simulink model "Workshop_as_sim_part2"  (Simulink 9.3)
settings: Solver=ode1  StartTime=0.0  StopTime=50  FixedStep=0.001  RelTol=1e-3  EnableMultiTasking=on
PostLoadFcn:
  | qc_set_target_type(getConfigSet(bdroot, 'QUARC Default Target Configuration'));
undefined symbols (not defined in the file or in its folder): actuator_pnoise_pow, actuator_tf_den, actuator_tf_num, anom_set_size, HIL, input_delay_length, qc_get_step_size, tire_mnoise_pow, use_actuator_pnoise, use_input_delay, use_roadpos_anomalies, use_roadpos_noise, use_tire_mnoise, use_vb_mnoise, vb_mnoise_pow
libraries: quarc_library x8, simulink x6, commrandsrc3 x1
settings Model: Creator=DCrymble  LastModifiedBy=jxs210080  SimulationMode=external  ExtModeTrigDuration=50000
settings SolverCC: PositivePriorityOrder=on
settings DataIOCC: LimitDataPoints=on
settings OptimizationCC: ExpressionDepthLimit=2147483647  InitFltsAndDblsToZero=on  LifeSpan=auto
settings DebuggingCC: SaveWithParameterizedLinksMsg=none  SolverPrmCheckMsg=warning  MultiTaskDSMMsg=warning  MultiTaskCondExecSysMsg=none  StateNameClashWarn=warning
settings RTWCC: SystemTargetFile=quarc_win64.tlc  TemplateMakefile=quarc_default_tmf  Description=QUARC Win64 Target
settings STFCustomTargetCC: TargetPreCompLibLocation=C:\PROGRA~3\QUARC\lib\2019a\win64\release  ConcurrentExecutionCompliant=on  SystemTargetFile=quarc_win64.tlc
settings GRTTargetCC: TargetPreCompLibLocation=C:\PROGRA~3\QUARC\lib\2019a\win64\release  ParMdlRefBuildCompliant=off  CompOptLevelCompliant=off  MatFileLogging=off  CPPClassGenCompliant=off  UseToolchainInfoCompliant=off  ExtMode=on  ExtModeMexFile=quarc_comm
settings ConfigComp: CovHtmlReporting=off

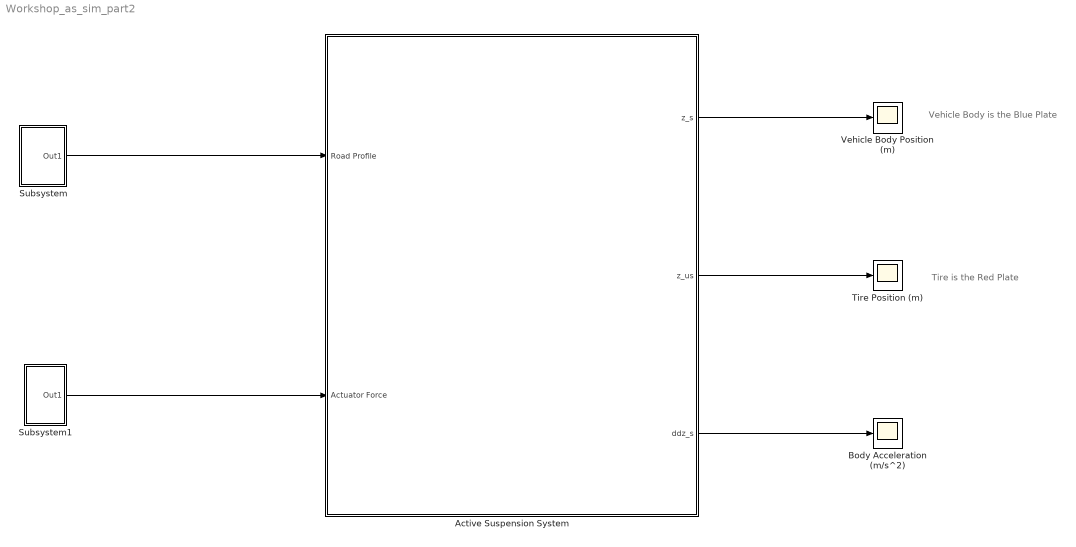
== system Workshop_as_sim_part2 ==
  note: Vehicle Body is the Blue Plate
  note: Tire is the Red Plate
  Active Suspension System : Subsystem
      mask Display: image('icon.png');
  Body Acceleration (m/s^2) : Scope
  Subsystem : Subsystem
  Subsystem1 : Subsystem
  Tire Position (m) : Scope
  Vehicle Body Position (m) : Scope
  wires:
  Active Suspension System/3(ddz_s) -> Body Acceleration (m/s^2)/1
  Active Suspension System/2(z_us) -> Tire Position (m)/1
  Active Suspension System/1(z_s) -> Vehicle Body Position (m)/1
  Subsystem/1(Out1) -> Active Suspension System/1(Road Profile)
  Subsystem1/1(Out1) -> Active Suspension System/2(Actuator Force)

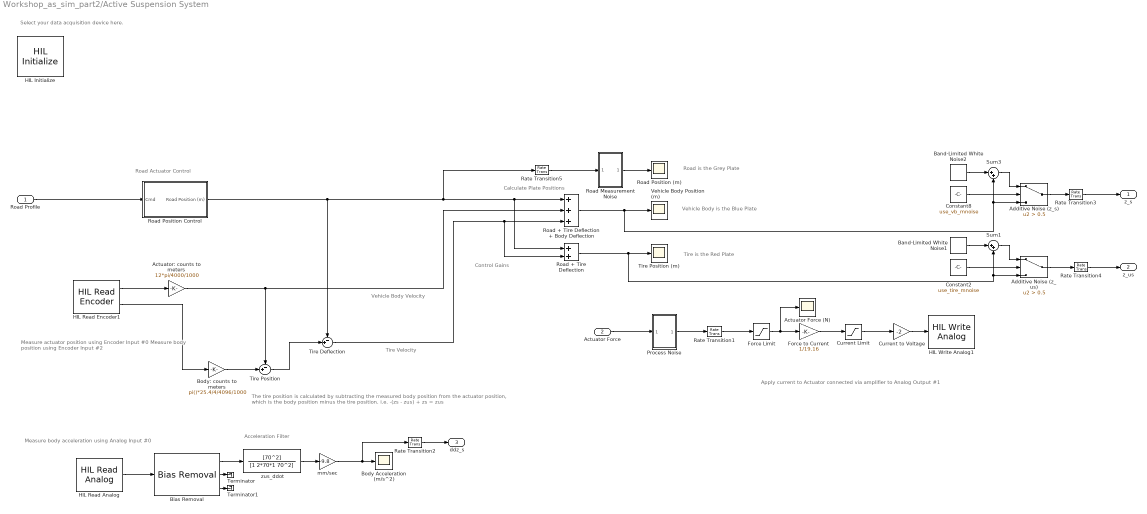
== system Workshop_as_sim_part2/Active Suspension System ==
  note: Measure actuator position using Encoder Input  #0
      | Measure body position using Encoder Input #2
  note: Select your data acquisition device here.
  note: Control Gains
  note: Vehicle Body Velocity
  note: Tire Velocity
  note: Road Actuator Control
  note: Calculate Plate Positions
  note: Measure body acceleration using Analog Input #0
  note: Acceleration Filter
  note: Apply current to Actuator connected via amplifier to Analog Output #1
  note: Road is the Grey Plate
  note: Vehicle Body is the Blue Plate
  note: Tire is the Red Plate
  note: The tire position is calculated by subtracting the measured body position from
      | the actuator position, which is the body position minus the tire position.
      | i.e. -(zs - zus) + zs = zus
  Road Profile : Inport
  Actuator Force : Inport  Port=2
  Actuator Force (N) : Scope
  Actuator: counts to meters : Gain  Gain=12*pi/4000/1000
  Additive Noise (z_s) : Switch  Criteria=u2 > Threshold  Threshold=0.5
  Additive Noise (z_us) : Switch  Criteria=u2 > Threshold  Threshold=0.5
  Band-Limited White Noise1 : simulink/Sources/Band-Limited White Noise  Cov=[tire_mnoise_pow]  Ts=0.001  seed=[23341]
  Band-Limited White Noise2 : simulink/Sources/Band-Limited White Noise  Cov=[vb_mnoise_pow]  Ts=0.001  seed=[23341]
  Bias Removal : quarc_library/Discrete/Bias Removal  start_time=0  end_time=.099  switch_id=0  sample_time=qc_get_step_size
      settings: SourceProductName=QUARC Targets
  Body Acceleration (m/s^2) : Scope
  Body: counts to meters : Gain  Gain=pi()*25.4/4/4096/1000
  Constant2 : Constant  Value=use_tire_mnoise
  Constant8 : Constant  Value=use_vb_mnoise
  Current Limit : Saturate  UpperLimit=5  LowerLimit=-5
  Current to Voltage : Gain  Gain=-2
  Force Limit : Saturate  UpperLimit=39.2  LowerLimit=-39.2
  Force to Current : Gain  Gain=1/19.16
  HIL Initialize : quarc_library/Data Acquisition/Generic/Configuration/HIL Initialize  Priority=-99  object_name=HIL-1  board_type=q8_usb  board_number=0  board_options=update_rate=normal;decimation=1  exclusive=off  active=off  hardware_clocks=[0:2]  clock_modes=[]  initial_clock_frequencies=[]  set_clock_params_at_start=off  set_clock_params_at_switch_in=off  set_clock_frequencies_at_start=off  set_clock_frequencies_at_switch_in=off  analog_input_channels=[0:7]  analog_input_configurations=[]  analog_input_maximums=10  analog_input_minimums=-10  set_analog_input_params_at_start=on  set_analog_input_params_at_switch_in=off  analog_output_channels=[0:7]  analog_output_maximums=10  analog_output_minimums=-10  initial_analog_outputs=[0]  final_analog_outputs=[0]  watchdog_analog_outputs=0  set_analog_output_params_at_start=on  set_analog_output_params_at_switch_in=off  set_analog_outputs_at_start=on  set_analog_outputs_at_switch_in=off  set_analog_outputs_at_terminate=on  set_analog_outputs_at_switch_out=off  set_analog_outputs_on_watchdog=off  digital_input_channels=[]  digital_output_channels=[0:4]  digital_output_configuration=[]  initial_digital_outputs=[0 0 0 0 1]  final_digital_outputs=[1 1 1 1 0]  watchdog_digital_outputs=[0]  set_digital_output_params_at_start=off  set_digital_output_params_at_switch_in=off  set_digital_outputs_at_start=on  set_digital_outputs_at_switch_in=on  set_digital_outputs_at_terminate=on  set_digital_outputs_at_switch_out=off  set_digital_outputs_on_watchdog=off  encoder_channels=[0:7]  quadrature=[4]  encoder_filter_frequency=[]  initial_encoder_counts=[0]  set_encoder_params_at_start=on  set_encoder_params_at_switch_in=off  set_encoder_counts_at_start=on  set_encoder_counts_at_switch_in=off  pwm_channels=[0:7]  pwm_modes=0  pwm_frequency=99.532799999999995e6/4095  pwm_configuration=[0]  pwm_alignment=[0]  pwm_polarity=[1]  pwm_leading_deadband=[0]  pwm_trailing_deadband=[0]  initial_pwm_outputs=[0]  final_pwm_outputs=[0]  watchdog_pwm_outputs=[0]  set_pwm_params_at_start=on  set_pwm_params_at_switch_in=off  set_pwm_outputs_at_start=on  set_pwm_outputs_at_switch_in=off  set_pwm_outputs_at_terminate=on  set_pwm_outputs_at_switch_out=off  set_pwm_outputs_on_watchdog=off  other_output_channels=[]  initial_other_outputs=[]  final_other_outputs=[]  watchdog_other_outputs=[]  set_other_outputs_at_start=off  set_other_outputs_at_switch_in=off  set_other_outputs_at_terminate=off  set_other_outputs_at_switch_out=off  set_other_outputs_on_watchdog=off
  HIL Read Analog : quarc_library/Data Acquisition/Generic/Immediate I//O/HIL Read Analog  object_name=HIL-1  channels=0  sample_time=qc_get_step_size  active=on  vector_output=off
  HIL Read Encoder1 : quarc_library/Data Acquisition/Generic/Immediate I//O/HIL Read Encoder  object_name=HIL-1  channels=[0, 2]  sample_time=qc_get_step_size  active=on  vector_output=off  data_type_mode=Inherit via back propagation  data_type=double
  HIL Write Analog1 : quarc_library/Data Acquisition/Generic/Immediate I//O/HIL Write Analog  object_name=HIL-1  channels=0  sample_time=-1  active=off  vector_input=on
  "Process Noise " : Subsystem
  Rate Transition1 : RateTransition  OutPortSampleTime=0.1
  Rate Transition{2..5} (4 alike) : RateTransition  OutPortSampleTime=0.01
  Road + Tire Deflection : Sum  Inputs=2  SaturateOnIntegerOverflow=on  InputSameDT=on  OutDataTypeStr=Inherit: Same as first input
  Road + Tire Deflection + Body Deflection : Sum  Inputs=3  SaturateOnIntegerOverflow=on  InputSameDT=on  OutDataTypeStr=Inherit: Same as first input
  Road Measurement Noise : Subsystem
  Road Position (m) : Scope
  Road Position Control : Subsystem
  Sum1 : Sum  Inputs=|++
  Sum3 : Sum  Inputs=|++
  Terminator : Terminator
  Terminator1 : Terminator
  Tire Deflection : Sum  Inputs=-+|
  Tire Position : Sum  Inputs=-+|
  Tire Position (m) : Scope
  Vehicle Body Position (m) : Scope
  mm/sec : Gain  Gain=-9.8
  zus_ddot : TransferFcn  Numerator=[70^2]  Denominator=[1 2*70*1 70^2]
  z_s : Outport
  z_us : Outport  Port=2
  ddz_s : Outport  Port=3
  wires:
  HIL Read Encoder1/1 -> Actuator: counts to meters/1
  Tire Deflection/1 -> Road + Tire Deflection + Body Deflection/3, Road + Tire Deflection/2
  HIL Read Encoder1/2 -> Body: counts to meters/1
  Body: counts to meters/1 -> Tire Position/2
  Road Position Control/1(Road Position (m)) -> Tire Deflection/1, Road + Tire Deflection + Body Deflection/1, Road + Tire Deflection/1, Rate Transition5/1
  Tire Position/1 -> Tire Deflection/2
  Bias Removal/2 -> Terminator/1
  Current to Voltage/1 -> HIL Write Analog1/1
  Force to Current/1 -> Current Limit/1
  Road Profile/1 -> Road Position Control/1(Cmd)
  Force Limit/1 -> Actuator Force (N)/1, Force to Current/1
  zus_ddot/1 -> mm/sec/1
  mm/sec/1 -> Rate Transition2/1, Body Acceleration (m/s^2)/1
  Bias Removal/1 -> zus_ddot/1
  Current Limit/1 -> Current to Voltage/1
  HIL Read Analog/1 -> Bias Removal/1
  Bias Removal/3 -> Terminator1/1
  Actuator Force/1 -> "Process Noise "/1(In1)
  Rate Transition2/1 -> ddz_s/1
  Rate Transition4/1 -> z_us/1
  Rate Transition3/1 -> z_s/1
  Rate Transition1/1 -> Force Limit/1
  Road + Tire Deflection + Body Deflection/1 -> Vehicle Body Position (m)/1, Sum3/2, Additive Noise (z_s)/3
  Additive Noise (z_s)/1 -> Rate Transition3/1
  Sum3/1 -> Additive Noise (z_s)/1
  Band-Limited White Noise2/1 -> Sum3/1
  Constant8/1 -> Additive Noise (z_s)/2
  Constant2/1 -> Additive Noise (z_us)/2
  Band-Limited White Noise1/1 -> Sum1/1
  Sum1/1 -> Additive Noise (z_us)/1
  Additive Noise (z_us)/1 -> Rate Transition4/1
  Road + Tire Deflection/1 -> Sum1/2, Additive Noise (z_us)/3, Tire Position (m)/1
  Actuator: counts to meters/1 -> Tire Position/1, Road + Tire Deflection + Body Deflection/2
  Road Measurement Noise/1(Out1) -> Road Position (m)/1
  "Process Noise "/1(Out1) -> Rate Transition1/1
  Rate Transition5/1 -> Road Measurement Noise/1(In1)

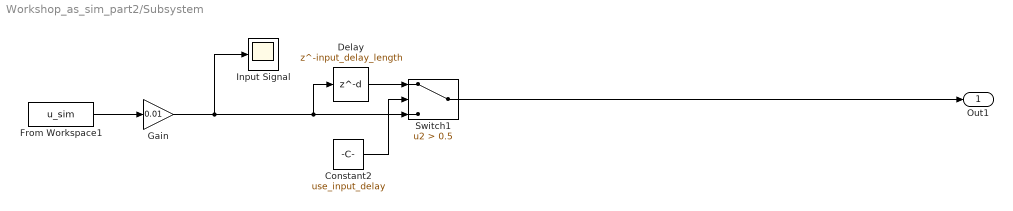
== system Workshop_as_sim_part2/Subsystem ==
  Constant2 : Constant  Value=use_input_delay
  Delay : Delay  DelayLength=input_delay_length
  From Workspace1 : FromWorkspace  VariableName=u_sim  SampleTime=0.01
  Gain : Gain  Gain=0.01
  Input Signal : Scope
  Switch1 : Switch  Criteria=u2 > Threshold  Threshold=0.5
  Out1 : Outport
  wires:
  Switch1/1 -> Out1/1
  From Workspace1/1 -> Gain/1
  Gain/1 -> Input Signal/1, Delay/1, Switch1/3
  Delay/1 -> Switch1/1
  Constant2/1 -> Switch1/2

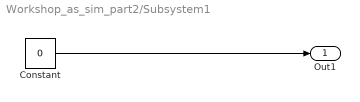
== system Workshop_as_sim_part2/Subsystem1 ==
  Constant : Constant  Value=0
  Out1 : Outport
  wires:
  Constant/1 -> Out1/1

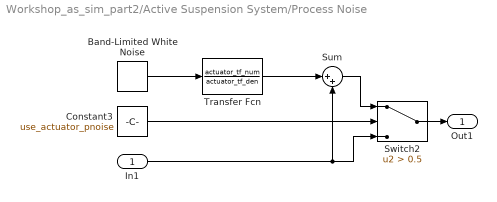
== system Workshop_as_sim_part2/Active Suspension System/Process Noise  ==
  In1 : Inport
  Band-Limited White Noise : simulink/Sources/Band-Limited White Noise  Cov=[actuator_pnoise_pow]  Ts=0.001  seed=[23341]
  Constant3 : Constant  Value=use_actuator_pnoise
  Sum : Sum  Inputs=|++
  Switch2 : Switch  Criteria=u2 > Threshold  Threshold=0.5
  Transfer Fcn : TransferFcn  Numerator=actuator_tf_num  Denominator=actuator_tf_den
  Out1 : Outport
  wires:
  Band-Limited White Noise/1 -> Transfer Fcn/1
  In1/1 -> Switch2/3, Sum/2
  Transfer Fcn/1 -> Sum/1
  Constant3/1 -> Switch2/2
  Sum/1 -> Switch2/1
  Switch2/1 -> Out1/1

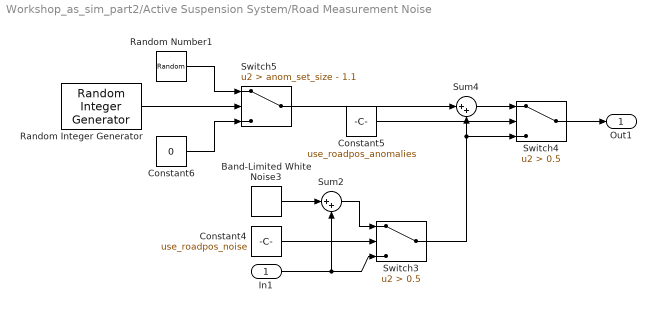
== system Workshop_as_sim_part2/Active Suspension System/Road Measurement Noise ==
  In1 : Inport
  Band-Limited White Noise3 : simulink/Sources/Band-Limited White Noise  Cov=roadpos_noise_pow  Ts=0.01  seed=[23341]
  Constant4 : Constant  Value=use_roadpos_noise
  Constant5 : Constant  Value=use_roadpos_anomalies
  Constant6 : Constant  Value=0
  Random Number1 : RandomNumber  Variance=100  SampleTime=0.01
  Random Integer Generator : commrandsrc3/Random Integer Generator  SetSize=anom_set_size  SeedSource=Auto  Seed=0  SampleTime=0.01  SamplesPerFrame=1  OutputDataType=double  SimulateUsing=Interpreted execution
      settings: SourceProductName=Communications Toolbox
  Sum2 : Sum  Inputs=|++
  Sum4 : Sum  Inputs=|++
  Switch3 : Switch  Criteria=u2 > Threshold  Threshold=0.5
  Switch4 : Switch  Criteria=u2 > Threshold  Threshold=0.5
  Switch5 : Switch  Criteria=u2 > Threshold  Threshold=anom_set_size - 1.1
  Out1 : Outport
  wires:
  Band-Limited White Noise3/1 -> Sum2/1
  Switch5/1 -> Sum4/1
  Random Integer Generator/1 -> Switch5/2
  Constant4/1 -> Switch3/2
  Constant5/1 -> Switch4/2
  Random Number1/1 -> Switch5/1
  Sum4/1 -> Switch4/1
  Switch3/1 -> Switch4/3, Sum4/2
  Constant6/1 -> Switch5/3
  In1/1 -> Sum2/2, Switch3/3
  Sum2/1 -> Switch3/1
  Switch4/1 -> Out1/1

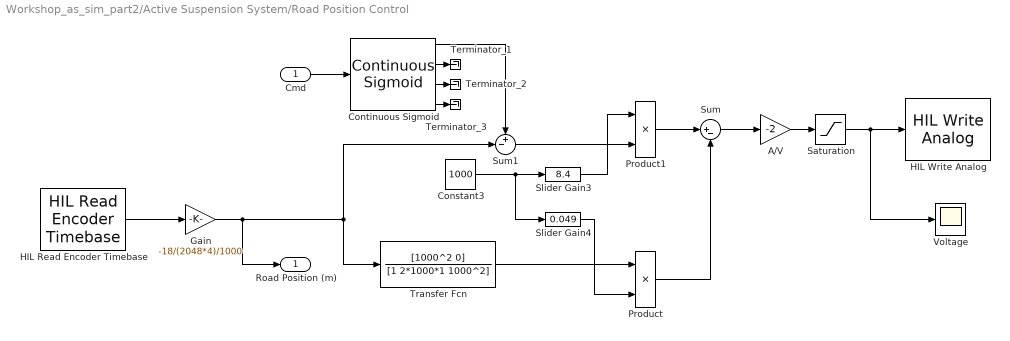
== system Workshop_as_sim_part2/Active Suspension System/Road Position Control ==
  Cmd : Inport
  A/V : Gain  Gain=-2
  Constant3 : Constant  Value=1000
  Continuous Sigmoid : quarc_library/Sources/Sigmoids/Continuous Sigmoid  params_source=Internal (dialog parameters)  max_velocity=.6/3  max_acceleration=20  initial_position=0  initial_velocity=0  hold_off=0.5  input_sample_time=-1  output_sample_time=qc_get_step_size
      settings: SourceProductName=QUARC Targets
  Gain : Gain  Gain=-18/(2048*4)/1000
  HIL Read Encoder Timebase : quarc_library/Data Acquisition/Generic/Timebases/HIL Read Encoder Timebase  object_name=HIL-1  clock=[0]  channels=1  samples_in_buffer=max(ceil(1/qc_get_step_size), 1)  active=on  vector_output=on  data_type_mode=Inherit via back propagation  data_type=double
  HIL Write Analog : quarc_library/Data Acquisition/Generic/Immediate I//O/HIL Write Analog  object_name=HIL-1  channels=1  sample_time=-1  active=off  vector_input=on
  Product : Product  RndMeth=Zero
  Product1 : Product  RndMeth=Zero
  Saturation : Saturate  UpperLimit=10  LowerLimit=-10
  Slider Gain3 : simulink/Math Operations/Slider Gain  gain=8.4  low=0  high=70
  Slider Gain4 : simulink/Math Operations/Slider Gain  gain=0.049  low=0  high=0.1
  Sum : Sum  Inputs=|+-
  Sum1 : Sum  Inputs=+-|
  Terminator_1 : Terminator
  Terminator_2 : Terminator
  Terminator_3 : Terminator
  Transfer Fcn : TransferFcn  Numerator=[1000^2 0]  Denominator=[1 2*1000*1 1000^2]
  Voltage : Scope
  Road Position (m) : Outport
  wires:
  A/V/1 -> Saturation/1
  Constant3/1 -> Slider Gain4/1, Slider Gain3/1
  HIL Read Encoder Timebase/1 -> Gain/1
  Saturation/1 -> HIL Write Analog/1, Voltage/1
  Sum/1 -> A/V/1
  Gain/1 -> Road Position (m)/1, Transfer Fcn/1, Sum1/2
  Transfer Fcn/1 -> Product/1
  Slider Gain3/1 -> Product1/1
  Sum1/1 -> Product1/2
  Product1/1 -> Sum/1
  Slider Gain4/1 -> Product/2
  Product/1 -> Sum/2
  Continuous Sigmoid/2 -> Terminator_1/1
  Continuous Sigmoid/3 -> Terminator_2/1
  Continuous Sigmoid/4 -> Terminator_3/1
  Continuous Sigmoid/1 -> Sum1/1
  Cmd/1 -> Continuous Sigmoid/1
